simulink model "hardware_stabilizing_controller"  (R2023a)
settings: Solver=VariableStepAuto  StartTime=0.0  StopTime=10.0  RelTol=1e-3
undefined symbols (not defined in the file): R_1_front, R_1_side
libraries: legoev3lib x6
settings Model: Creator=morit  LastModifiedBy=morit

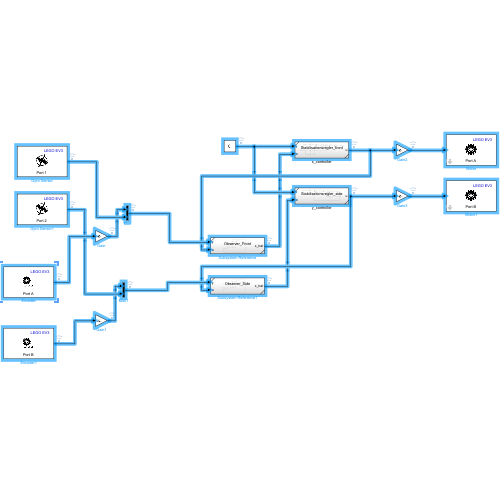
[thumbnail: Simulink's stored preview of the top-level diagram]
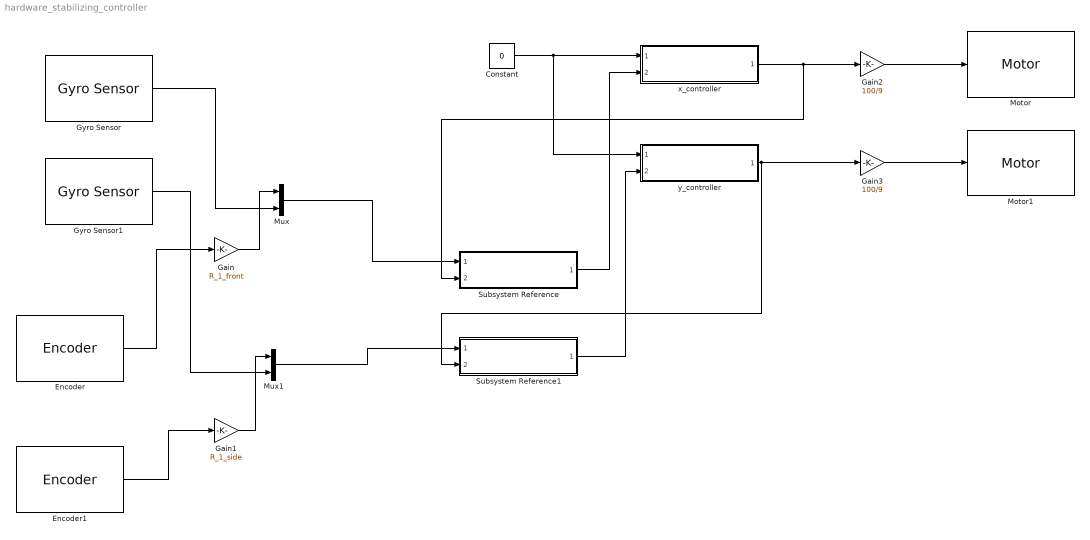
== system hardware_stabilizing_controller ==
  Constant : Constant  Value=0
  Encoder : legoev3lib/Encoder  portNumber=A  opMode=Reset at each sample time  sampleTime=0.1
  Encoder1 : legoev3lib/Encoder  portNumber=B  opMode=Reset at each sample time  sampleTime=0.1
  Gain : Gain  Gain=R_1_front
  Gain1 : Gain  Gain=R_1_side
  Gain2 : Gain  Gain=100/9
  Gain3 : Gain  Gain=100/9
  Gyro Sensor : legoev3lib/Gyro Sensor  portNumber=1  sampleTime=0.1
  Gyro Sensor1 : legoev3lib/Gyro Sensor  portNumber=2  sampleTime=0.1
  Motor : legoev3lib/Motor  sportNumber=A  sstopAction=Brake
  Motor1 : legoev3lib/Motor  sportNumber=B  sstopAction=Brake
  Mux : Mux  Inputs=2
  Mux1 : Mux  Inputs=2
  Subsystem Reference : Subsystem  ReferencedSubsystem=Observer_Front
  Subsystem Reference1 : Subsystem  ReferencedSubsystem=Observer_Side
  x_controller : Subsystem  ReferencedSubsystem=Stabilisationsregler_front
  y_controller : Subsystem  ReferencedSubsystem=Stabilisationsregler_side
  wires:
  Constant/1 -> y_controller/1, x_controller/1
  x_controller/1 -> Subsystem Reference/2, Gain2/1
  y_controller/1 -> Subsystem Reference1/2, Gain3/1
  Subsystem Reference/1 -> x_controller/2
  Subsystem Reference1/1 -> y_controller/2
  Gyro Sensor/1 -> Mux/2
  Gyro Sensor1/1 -> Mux1/2
  Encoder1/1 -> Gain1/1
  Encoder/1 -> Gain/1
  Gain/1 -> Mux/1
  Gain1/1 -> Mux1/1
  Mux1/1 -> Subsystem Reference1/1
  Mux/1 -> Subsystem Reference/1
  Gain2/1 -> Motor/1
  Gain3/1 -> Motor1/1
